simulink model "model_reg_silnik2014a"  (R2014a)
settings: Solver=ode4  StartTime=0.0  StopTime=20  FixedStep=0.001  RelTol=1e-3
values from neighbouring files (symbols this model uses):
  limitT = 0.05    [dane.m]
  lin = 1    [dane.m]
  mc = 0.741    [dane.m]
  mw = 1.155    [dane.m]
  omega = (x0(9)/g)^0.5    [dane.m]
  p = 60    [dane.m]
  reg_PD = 0    [dane.m]
  x0 = [0   0   0    0   0   0    0   0   0.250   0]'    [dane.m]
undefined symbols (not defined in the file or in its folder): A, B, C, D
libraries: simulink x3
settings Model: CovModelRefEnable=off  CovSFcnEnable=on  Creator=Maciek  LastModifiedBy=Maciek
settings SolverCC: AlgebraicLoopSolver=LineSearch
settings DataIOCC: LimitDataPoints=off  SaveFormat=StructureWithTime
settings DebuggingCC: MergeDetectMultiDrivingBlocksExec=error  SolverPrmCheckMsg=none  FrameProcessingCompatibilityMsg=error
settings HardwareCC: ProdBitPerPointer=64  ProdLargestAtomicFloat=Float  ProdIntDivRoundTo=Zero  ProdEndianess=LittleEndian  ProdHWDeviceType=Specified
settings ModelReferenceCC: PropagateSignalLabelsOutOfModel=on

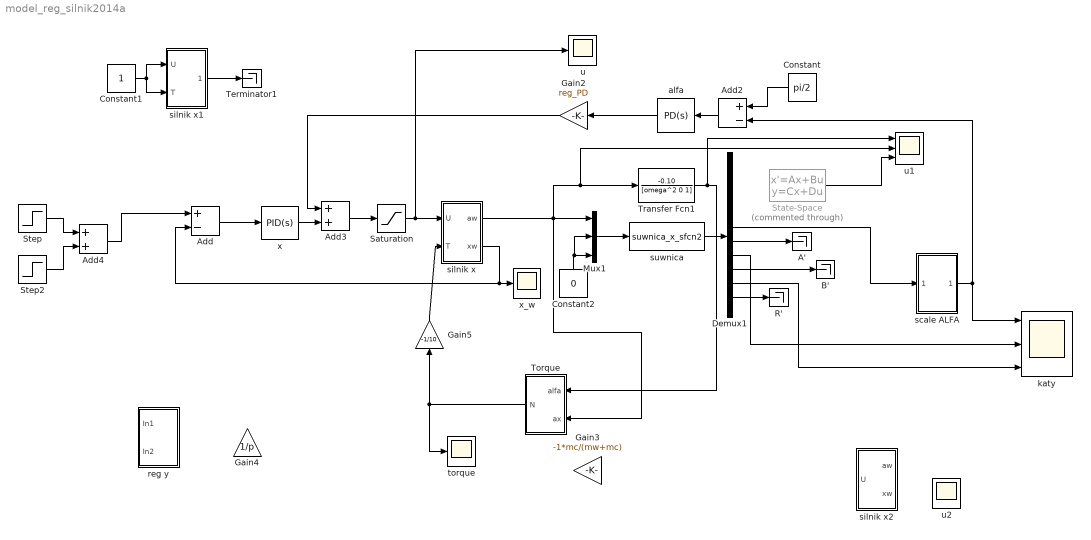
== system model_reg_silnik2014a ==
  A' : Terminator
  Add : Sum  Inputs=+-
  Add2 : Sum  Inputs=+-
  Add3 : Sum
  Add4 : Sum
  B' : Terminator
  Constant : Constant  Value=pi/2
  Constant1 : Constant
  Constant2 : Constant  Value=0
  Demux1 : Demux  Outputs=10
  Gain2 : Gain  Gain=reg_PD
  Gain3 : Gain  Gain=-1*mc/(mw+mc)
  Gain4 : Gain  Gain=1/p
  Gain5 : Gain  Gain=-1/10
  Mux1 : Mux  Inputs=3
  R' : Terminator
  Saturation : Saturate  UpperLimit=1  LowerLimit=-1
  State-Space : StateSpace  Commented=through  A=A  B=B  C=C  D=D  X0=[0 0]
  Step : Step  After=0.2  SampleTime=0
  Step2 : Step  Time=40  After=-0.7  SampleTime=0
  Terminator1 : Terminator
  "Torque " : Subsystem
  Transfer Fcn1 : TransferFcn  Numerator=-0.10  Denominator=[omega^2 0 1]
  alfa : simulink/Continuous/PID Controller  Controller=PD  TimeDomain=Continuous-time  SampleTime=-1  IntegratorMethod=Forward Euler  FilterMethod=Forward Euler  Form=Parallel  UseFilter=on  ControllerParametersSource=internal  P=10  I=0.015  D=0.5  N=100  InitialConditionSource=internal  InitialConditionForIntegrator=0  InitialConditionForFilter=0  ExternalReset=none  LimitOutput=on  UpperSaturationLimit=1  LowerSaturationLimit=-1  LinearizeAsGain=on  AntiWindupMode=none  Kb=1  TrackingMode=off  Kt=1  PParamMin=[]  PParamMax=[]  IParamMin=[]  IParamMax=[]  DParamMin=[]  DParamMax=[]  NParamMin=[]  NParamMax=[]  KbParamMin=[]  KbParamMax=[]  KtParamMin=[]  KtParamMax=[]  POutMin=[]  POutMax=[]  IOutMin=[]  IOutMax=[]  DOutMin=[]  DOutMax=[]  NOutMin=[]  NOutMax=[]  KbOutMin=[]  KbOutMax=[]  KtOutMin=[]  KtOutMax=[]  IntegratorOutMin=[]  IntegratorOutMax=[]  FilterOutMin=[]  FilterOutMax=[]  SumOutMin=[]  SumOutMax=[]  SumI1OutMin=[]  SumI1OutMax=[]  SumI2OutMin=[]  SumI2OutMax=[]  SumI3OutMin=[]  SumI3OutMax=[]  SumDOutMin=[]  SumDOutMax=[]  SaturationOutMin=[]  SaturationOutMax=[]  IntegratorContinuousStateAttributes=''  IntegratorStateMustResolveToSignalObject=off  IntegratorRTWStateStorageClass=Auto  FilterContinuousStateAttributes=''  FilterStateMustResolveToSignalObject=off  FilterRTWStateStorageClass=Auto  DifferentiatorICPrevScaledInput=0  DifferentiatorOutMin=[]  DifferentiatorOutMax=[]
  katy : Scope  NumInputPorts=3
      settings: TimeRange=auto  MaxDataPoints=5000  SaveName=angle  YMin=1.26843~-1.00000~0.15  YMax=1.87237~1.00000~0.35  SampleTime=-1
  reg y : Subsystem
  scale ALFA : Subsystem
  silnik x : Subsystem
  silnik x1 : Subsystem
  silnik x2 : Subsystem
  suwnica : S-Function  FunctionName=suwnica_x_sfcn2  Parameters=x0  SFunctionDeploymentMode=off  EnableBusSupport=off
  torque : Scope
      settings: TimeRange=auto  MaxDataPoints=5000  SaveToWorkspace=off  YMin=-3.19541  YMax=1.34336  SampleTime=-1
  u : Scope
      settings: TimeRange=auto  MaxDataPoints=5000  SaveName=ster  YMin=-0.125  YMax=1.125  SampleTime=-1
  u1 : Scope  NumInputPorts=3
      settings: TimeRange=auto  MaxDataPoints=5000  SaveName=ster1  YMin=-0.28047~-1.52549~-0.29449  YMax=0.29302~8.05285~0.30043  SampleTime=-1
  u2 : Scope
      settings: TimeRange=auto  MaxDataPoints=5000  YMin=-0.02449  YMax=0.22039  SampleTime=-1
  x : simulink/Continuous/PID Controller  Controller=PID  TimeDomain=Continuous-time  SampleTime=-1  IntegratorMethod=Forward Euler  FilterMethod=Forward Euler  Form=Parallel  UseFilter=on  ControllerParametersSource=internal  P=10  I=0.005  D=2  N=100  InitialConditionSource=internal  InitialConditionForIntegrator=0  InitialConditionForFilter=0  ExternalReset=none  LimitOutput=on  UpperSaturationLimit=1  LowerSaturationLimit=-1  LinearizeAsGain=on  AntiWindupMode=none  Kb=1  TrackingMode=off  Kt=1  PParamMin=[]  PParamMax=[]  IParamMin=[]  IParamMax=[]  DParamMin=[]  DParamMax=[]  NParamMin=[]  NParamMax=[]  KbParamMin=[]  KbParamMax=[]  KtParamMin=[]  KtParamMax=[]  POutMin=[]  POutMax=[]  IOutMin=[]  IOutMax=[]  DOutMin=[]  DOutMax=[]  NOutMin=[]  NOutMax=[]  KbOutMin=[]  KbOutMax=[]  KtOutMin=[]  KtOutMax=[]  IntegratorOutMin=[]  IntegratorOutMax=[]  FilterOutMin=[]  FilterOutMax=[]  SumOutMin=[]  SumOutMax=[]  SumI1OutMin=[]  SumI1OutMax=[]  SumI2OutMin=[]  SumI2OutMax=[]  SumI3OutMin=[]  SumI3OutMax=[]  SumDOutMin=[]  SumDOutMax=[]  SaturationOutMin=[]  SaturationOutMax=[]  IntegratorContinuousStateAttributes=''  IntegratorStateMustResolveToSignalObject=off  IntegratorRTWStateStorageClass=Auto  FilterContinuousStateAttributes=''  FilterStateMustResolveToSignalObject=off  FilterRTWStateStorageClass=Auto  DifferentiatorICPrevScaledInput=0  DifferentiatorOutMin=[]  DifferentiatorOutMax=[]
  "x_w " : Scope
      settings: TimeRange=auto  MaxDataPoints=5000  SaveName=newX  YMin=-0.02442  YMax=0.21979  SampleTime=-1
  wires:
  Mux1/1 -> suwnica/1
  Constant2/1 -> Mux1/2, Mux1/3
  Demux1/10 -> R'/1
  Demux1/8 -> B'/1
  Demux1/7 -> katy/2
  Demux1/9 -> katy/3
  Demux1/6 -> A'/1
  suwnica/1 -> Demux1/1
  scale ALFA/1(Out1) -> Add2/2, katy/1
  Add/1 -> x/1
  Add2/1 -> alfa/1
  Constant/1 -> Add2/1
  alfa/1 -> Gain2/1
  x/1 -> Add3/2
  Saturation/1 -> u/1, silnik x/1(U)
  Gain2/1 -> Add3/1
  silnik x/1(aw) -> Mux1/1, "Torque "/2(ax), u1/2, Transfer Fcn1/1
  silnik x/2(xw) -> Add/2, "x_w "/1
  silnik x1/1(Out1) -> Terminator1/1
  Constant1/1 -> silnik x1/1(U), silnik x1/2(T)
  Add4/1 -> Add/1
  Step/1 -> Add4/1
  Step2/1 -> Add4/2
  Transfer Fcn1/1 -> "Torque "/1(alfa), u1/1
  Add3/1 -> Saturation/1
  Demux1/5 -> scale ALFA/1(In1)
  State-Space/1 -> u1/3
  Gain5/1 -> silnik x/2(T)
  "Torque "/1(N) -> Gain5/1, torque/1

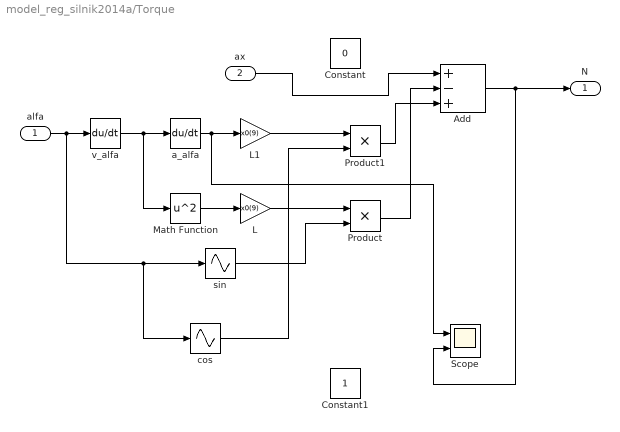
== system model_reg_silnik2014a/Torque  ==
  alfa : Inport
  ax : Inport  Port=2
  Add : Sum  Inputs=+-+
  Constant : Constant  Value=0
  Constant1 : Constant
  L : Gain  Gain=x0(9)
  "L1 " : Gain  Gain=x0(9)
  Math Function : Math  Operator=square  SaturateOnIntegerOverflow=on
  Product : Product
  Product1 : Product
  Scope : Scope  NumInputPorts=2
      settings: TimeRange=auto  MaxDataPoints=5000  SaveToWorkspace=off  SaveName=ScopeData  YMin=-34.60443~-3.28476  YMax=15.82675~4.86648  SampleTime=-1
  a_alfa : Derivative
  cos : Sin  TimeSource=Use external signal  Phase=pi/2  SampleTime=0
  sin : Sin  TimeSource=Use external signal  SampleTime=0
  v_alfa : Derivative
  N : Outport
  wires:
  a_alfa/1 -> Scope/1, "L1 "/1
  v_alfa/1 -> Math Function/1, a_alfa/1
  Math Function/1 -> L/1
  L/1 -> Product/1
  Product/1 -> Add/2
  alfa/1 -> cos/1, sin/1, v_alfa/1
  "L1 "/1 -> Product1/1
  Product1/1 -> Add/3
  Add/1 -> Scope/2, N/1
  cos/1 -> Product1/2
  ax/1 -> Add/1
  sin/1 -> Product/2

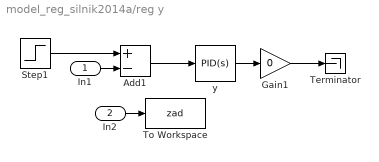
== system model_reg_silnik2014a/reg y ==
  In1 : Inport
  In2 : Inport  Port=2
  Add1 : Sum  Inputs=+-
  Gain1 : Gain  Gain=0
  Step1 : Step  After=0  SampleTime=0
  Terminator : Terminator
  To Workspace : ToWorkspace  VariableName=zad  SaveFormat=Timeseries  SampleTime=-1
  y : simulink/Continuous/PID Controller  Controller=PID  TimeDomain=Continuous-time  SampleTime=-1  IntegratorMethod=Forward Euler  FilterMethod=Forward Euler  Form=Parallel  UseFilter=on  ControllerParametersSource=internal  P=250  I=0.002  D=1  N=100  InitialConditionSource=internal  InitialConditionForIntegrator=0  InitialConditionForFilter=0  ExternalReset=none  LimitOutput=on  UpperSaturationLimit=20  LowerSaturationLimit=-20  LinearizeAsGain=on  AntiWindupMode=none  Kb=1  TrackingMode=off  Kt=1  PParamMin=[]  PParamMax=[]  IParamMin=[]  IParamMax=[]  DParamMin=[]  DParamMax=[]  NParamMin=[]  NParamMax=[]  KbParamMin=[]  KbParamMax=[]  KtParamMin=[]  KtParamMax=[]  POutMin=[]  POutMax=[]  IOutMin=[]  IOutMax=[]  DOutMin=[]  DOutMax=[]  NOutMin=[]  NOutMax=[]  KbOutMin=[]  KbOutMax=[]  KtOutMin=[]  KtOutMax=[]  IntegratorOutMin=[]  IntegratorOutMax=[]  FilterOutMin=[]  FilterOutMax=[]  SumOutMin=[]  SumOutMax=[]  SumI1OutMin=[]  SumI1OutMax=[]  SumI2OutMin=[]  SumI2OutMax=[]  SumI3OutMin=[]  SumI3OutMax=[]  SumDOutMin=[]  SumDOutMax=[]  SaturationOutMin=[]  SaturationOutMax=[]  IntegratorContinuousStateAttributes=''  IntegratorStateMustResolveToSignalObject=off  IntegratorRTWStateStorageClass=Auto  FilterContinuousStateAttributes=''  FilterStateMustResolveToSignalObject=off  FilterRTWStateStorageClass=Auto  DifferentiatorICPrevScaledInput=0  DifferentiatorOutMin=[]  DifferentiatorOutMax=[]
  wires:
  In1/1 -> Add1/2
  In2/1 -> To Workspace/1
  y/1 -> Gain1/1
  Add1/1 -> y/1
  Step1/1 -> Add1/1
  Gain1/1 -> Terminator/1

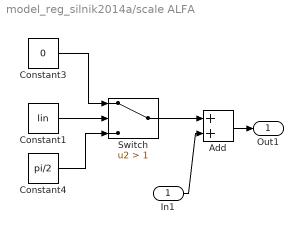
== system model_reg_silnik2014a/scale ALFA ==
  In1 : Inport
  Add : Sum  Inputs=2
  Constant1 : Constant  Value=lin
  Constant3 : Constant  Value=0
  Constant4 : Constant  Value=pi/2
  Switch : Switch  Criteria=u2 > Threshold  Threshold=1
  Out1 : Outport
  wires:
  Add/1 -> Out1/1
  In1/1 -> Add/2
  Constant4/1 -> Switch/3
  Constant3/1 -> Switch/1
  Switch/1 -> Add/1
  Constant1/1 -> Switch/2

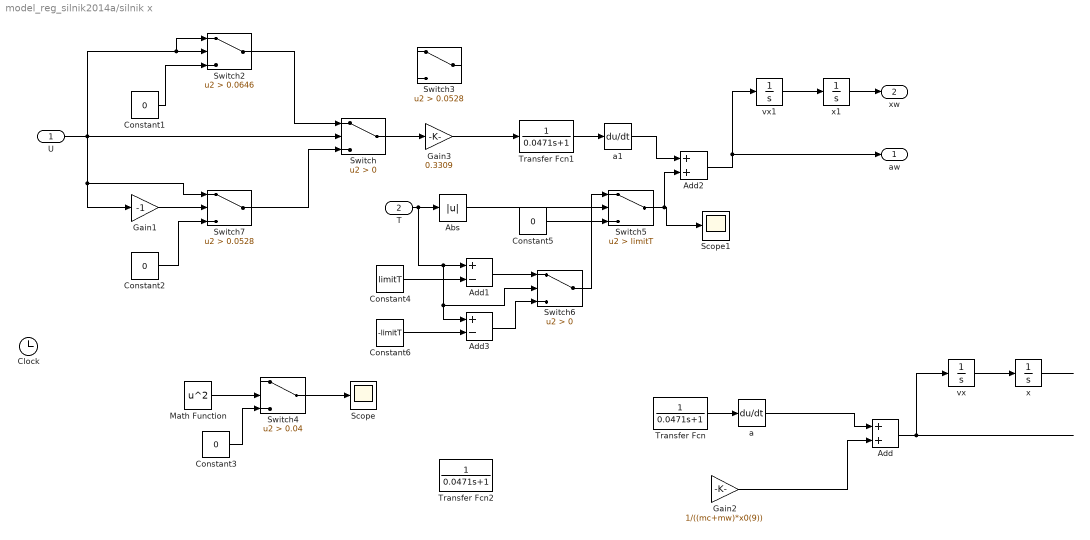
== system model_reg_silnik2014a/silnik x ==
  U : Inport
  T : Inport  Port=2
  Abs : Abs
  Add : Sum
  Add1 : Sum  Inputs=+-
  Add2 : Sum
  Add3 : Sum  Inputs=+-
  Clock : Clock
  Constant{1..3,5} (4 alike) : Constant  Value=0
  Constant4 : Constant  Value=limitT
  Constant6 : Constant  Value=-limitT
  Gain1 : Gain  Gain=-1
  Gain2 : Gain  Gain=1/((mc+mw)*x0(9))
  Gain3 : Gain  Gain=0.3309
  Math Function : Math  Operator=square  SaturateOnIntegerOverflow=on
  Scope : Scope
      settings: TimeRange=auto  MaxDataPoints=5000  SaveToWorkspace=off  YMin=-1.00000  YMax=1.00000  SampleTime=-1
  Scope1 : Scope
      settings: TimeRange=auto  MaxDataPoints=5000  SaveToWorkspace=off  SaveName=ScopeData2  YMin=-0.45032  YMax=0.28533  SampleTime=-1
  Switch : Switch  Criteria=u2 > Threshold
  Switch2 : Switch  Criteria=u2 > Threshold  Threshold=0.0646
  Switch3 : Switch  Criteria=u2 > Threshold  Threshold=0.0528
  Switch4 : Switch  Criteria=u2 > Threshold  Threshold=0.04
  Switch5 : Switch  Criteria=u2 > Threshold  Threshold=limitT
  Switch6 : Switch  Criteria=u2 > Threshold
  Switch7 : Switch  Criteria=u2 > Threshold  Threshold=0.0528
  Transfer Fcn : TransferFcn  Numerator=1  Denominator=[0.0471 1]
  Transfer Fcn1 : TransferFcn  Numerator=1  Denominator=[0.0471 1]
  Transfer Fcn2 : TransferFcn  Numerator=1  Denominator=[0.0471 1]
  a : Derivative
  a1 : Derivative
  vx : Integrator
  vx1 : Integrator
  x : Integrator
  x1 : Integrator
  aw : Outport
  xw : Outport  Port=2
  wires:
  Constant1/1 -> Switch2/3
  Switch2/1 -> Switch/1
  Constant2/1 -> Switch7/3
  U/1 -> Switch7/1, Gain1/1, Switch2/1, Switch2/2, Switch/2
  Switch7/1 -> Switch/3
  Gain1/1 -> Switch7/2
  Transfer Fcn/1 -> a/1
  ? -> Gain2/1
  a/1 -> Add/1
  Add/1 -> vx/1
  x/1 -> ?
  vx/1 -> x/1
  Gain2/1 -> Add/2
  ? -> Transfer Fcn/1
  Transfer Fcn1/1 -> a1/1
  x1/1 -> xw/1
  vx1/1 -> x1/1
  Gain3/1 -> Transfer Fcn1/1
  Add2/1 -> aw/1, vx1/1
  a1/1 -> Add2/1
  ? -> Math Function/1, Switch4/1
  Constant3/1 -> Switch4/3
  Math Function/1 -> Switch4/2
  Switch4/1 -> Scope/1
  Switch5/1 -> Add2/2, Scope1/1
  T/1 -> Add3/1, Switch6/2, Add1/1, Abs/1
  Abs/1 -> Switch5/2
  Constant4/1 -> Add1/2
  Constant5/1 -> Switch5/3
  Switch6/1 -> Switch5/1
  Add1/1 -> Switch6/1
  Constant6/1 -> Add3/2
  Add3/1 -> Switch6/3
  Switch/1 -> Gain3/1

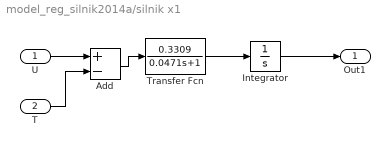
== system model_reg_silnik2014a/silnik x1 ==
  U : Inport
  T : Inport  Port=2
  Add : Sum  Inputs=+-
  Integrator : Integrator
  Transfer Fcn : TransferFcn  Numerator=0.3309  Denominator=[0.0471 1]
  Out1 : Outport
  wires:
  Transfer Fcn/1 -> Integrator/1
  Integrator/1 -> Out1/1
  Add/1 -> Transfer Fcn/1
  U/1 -> Add/1
  T/1 -> Add/2

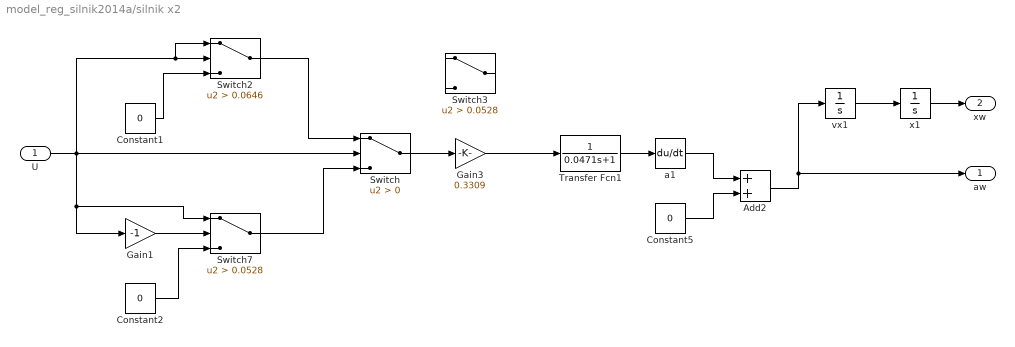
== system model_reg_silnik2014a/silnik x2 ==
  U : Inport
  Add2 : Sum
  Constant1 : Constant  Value=0
  Constant2 : Constant  Value=0
  Constant5 : Constant  Value=0
  Gain1 : Gain  Gain=-1
  Gain3 : Gain  Gain=0.3309
  Switch : Switch  Criteria=u2 > Threshold
  Switch2 : Switch  Criteria=u2 > Threshold  Threshold=0.0646
  Switch3 : Switch  Criteria=u2 > Threshold  Threshold=0.0528
  Switch7 : Switch  Criteria=u2 > Threshold  Threshold=0.0528
  Transfer Fcn1 : TransferFcn  Numerator=1  Denominator=[0.0471 1]
  a1 : Derivative
  vx1 : Integrator
  x1 : Integrator
  aw : Outport
  xw : Outport  Port=2
  wires:
  Constant1/1 -> Switch2/3
  Switch2/1 -> Switch/1
  Constant2/1 -> Switch7/3
  U/1 -> Switch7/1, Gain1/1, Switch2/1, Switch2/2, Switch/2
  Switch7/1 -> Switch/3
  Gain1/1 -> Switch7/2
  Transfer Fcn1/1 -> a1/1
  x1/1 -> xw/1
  vx1/1 -> x1/1
  Gain3/1 -> Transfer Fcn1/1
  Add2/1 -> aw/1, vx1/1
  a1/1 -> Add2/1
  Switch/1 -> Gain3/1
  Constant5/1 -> Add2/2
